simulink model "DirectedEvent2"  (R2020b)
settings: Solver=VariableStepAuto  StartTime=0.0  StopTime=0.1  RelTol=1e-3
settings Model: Creator=86188  LastModifiedBy=apple
settings DataIOCC: ReturnWorkspaceOutputs=off
settings DebuggingCC: ArithmeticOperatorsInVariantConditions=warning
settings SFSimCC: SimUseLocalCustomCode=off  CustomCodeUndefinedFunction=UseInterfaceOnly
settings RTWCC: RTWUseLocalCustomCode=off

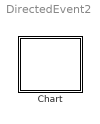
== system DirectedEvent2 ==
  Chart : Stateflow chart  TreatAsAtomicUnit=on

== stateflow chart DirectedEvent2/Chart ==
  settings: updateMethod=DISCRETE  sampleTime=0.1
  state AM
    state A [parallel]
      settings: executionOrder=1
      state A1
        en: fprintf("en_A1")
        ex: fprintf("ex_A1")
      state A2
        en: fprintf("en_A2")
        ex: fprintf("ex_A2")
      (default) -> AM.A.A1
      AM.A.A1 -> AM.A.A2 : [data==1]{B.E_one}
      AM.A.A2 -> AM.A.A1 : E_two
    state B [parallel]
      settings: executionOrder=2
      state A2
        en: fprintf("en_B2_A2")
        ex: fprintf("ex_B2_A2")
      state A1
        en: fprintf("en_B1_A1")
        ex: fprintf("ex_B1_A1")
      (default) -> AM.B.A1
      AM.B.A1 -> AM.B.A2 : E_one{C.E_one}
      AM.B.A2 -> AM.B.A1 : E_two{A.E_two}
    state C [parallel]
      settings: executionOrder=3
      state A2
        en: fprintf("en_C2_A2")
        ex: fprintf("ex_C2_A2")
      state A1
        en: fprintf("en_C1_A1")
        ex: fprintf("ex_C1_A1")
      (default) -> AM.C.A1
      AM.C.A1 -> AM.C.A2 : E_one
      AM.C.A2 -> AM.C.A1 : [data==1]{B.E_two}
  (default) -> AM : {data = 1;}
  data: data local double =1
  events: E_two local FUNCTION_CALL_EVENT; E_one local FUNCTION_CALL_EVENT; E_two local FUNCTION_CALL_EVENT; E_one local FUNCTION_CALL_EVENT
